simulink model "sim_1_twolink_joint_control_ideal"  (R2021a)
settings: Solver=ode15s  StartTime=0.0  StopTime=15  RelTol=1e-5  EnableMultiTasking=on
values from neighbouring files (symbols this model uses):
  b1 = 0.01    [sim_params.m]    (also in sim_params_force.m)
  b2 = 0.01    [sim_params.m]    (also in sim_params_force.m)
  D = [zeros(n); eye(n)]    [control_comparison_script.m]    (also in gen_twolink_ss.m = reshape([0.0,0.0,0.0,0.0,0.0,0.0,0.0,0.0],[4,2]))
  D_T_Q = D'*Q    [control_comparison_script.m]
  epsilon = 0.1    [control_comparison_script.m]
  g = 9.80665    [sim_params.m]    (also in sim_params_force.m)
  Kd1 = 2.5    [control_comparison_script.m]
  Kd1_grav = 2.5    [control_comparison_script.m]
  Kd1_inv = 12    [control_comparison_script.m]
  Kd1_robust = 7    [control_comparison_script.m]
  Kd2 = 0.5    [control_comparison_script.m]
  Kd2_grav = 0.5    [control_comparison_script.m]
  Kd2_inv = 15    [control_comparison_script.m]
  Kd2_robust = 35    [control_comparison_script.m]
  Klqr = lqr(A,B,Q,R)    [control_comparison_script.m]
  Kp1 = 30    [control_comparison_script.m]
  Kp1_grav = 15    [control_comparison_script.m]
  Kp1_inv = 25    [control_comparison_script.m]
  Kp1_robust = 25    [control_comparison_script.m]
  Kp2 = 7    [control_comparison_script.m]
  Kp2_grav = 3.5    [control_comparison_script.m]
  Kp2_inv = 50    [control_comparison_script.m]
  Kp2_robust = 45    [control_comparison_script.m]
  Kpp = place(A,B,p)    [control_comparison_script.m]
  L1x = 0.3    [sim_params.m]    (also in sim_params_force.m)
  L1y = 0.050    (= 0.05)    [sim_params.m]    (also in sim_params_force.m)
  L1z = 0.05    [sim_params.m]    (also in sim_params_force.m)
  L2x = 0.15    [sim_params.m]    (also in sim_params_force.m = 0.3)
  L2y = 0.05    [sim_params.m]    (also in sim_params_force.m)
  L2z = 0.05    [sim_params.m]    (also in sim_params_force.m)
  m1 = m1*1.25    [control_comparison_script.m]    (also in sim_params.m = 2.775; sim_params_force.m = 2.775)
  m2 = m2*1.25    [control_comparison_script.m]    (also in sim_params.m = 1.3875; sim_params_force.m = 2.775)
  N1 = 100    [control_comparison_script.m]
  N1_grav = 100    [control_comparison_script.m]
  N1_inv = 50    [control_comparison_script.m]
  N1_robust = 50    [control_comparison_script.m]
  N2 = 100    [control_comparison_script.m]
  N2_grav = 100    [control_comparison_script.m]
  N2_inv = 50    [control_comparison_script.m]
  N2_robust = 50    [control_comparison_script.m]
  rho = [1;1]    [control_comparison_script.m]
  theta1_0 = 0    [sim_params.m]    (also in sim_params_force.m = 1.57079632679)
  theta1_dot_0 = 0    [sim_params.m]    (also in sim_params_force.m)
  theta2_0 = 0    [sim_params.m]    (also in sim_params_force.m = -1.57079632679)
  theta2_dot_0 = 0    [sim_params.m]    (also in sim_params_force.m)
  Tsample = 0.001    [sim_params.m]    (also in sim_params_force.m)
undefined symbols (not defined in the file or in its folder): Kd, Ki, Kp, N, sigbuilder_block, X, Y, Z
libraries: pid_lib x12, sm_lib x11, nesl_utility x10, simulink_extras x8, spsFirstOrderFilterLib x4, dspmtrx3 x1
(part 3 of 3)

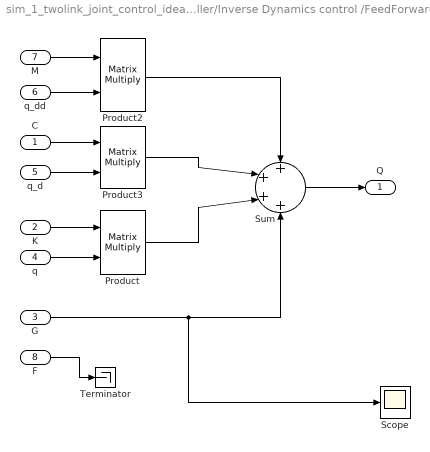
== system sim_1_twolink_joint_control_ideal/Controller/Inverse Dynamics control /FeedForward terms ==
  C : Inport
  K : Inport  Port=2
  G : Inport  Port=3
  q : Inport  Port=4
  q_d : Inport  Port=5
  q_dd : Inport  Port=6
  M : Inport  Port=7
  F : Inport  Port=8
  Product : Product  Multiplication=Matrix(*)
  Product2 : Product  Multiplication=Matrix(*)
  Product3 : Product  Multiplication=Matrix(*)
  Scope : Scope
  Sum : Sum  Inputs=+|+|+|+
  Terminator : Terminator
  Q : Outport
  wires:
  K/1 -> Product/1
  Product/1 -> Sum/3
  Product2/1 -> Sum/1
  Sum/1 -> Q/1
  C/1 -> Product3/1
  Product3/1 -> Sum/2
  M/1 -> Product2/1
  q_dd/1 -> Product2/2
  q/1 -> Product/2
  q_d/1 -> Product3/2
  F/1 -> Terminator/1
  G/1 -> Scope/1, Sum/4

== matlab function sim_1_twolink_joint_control_ideal/Controller/Robust control /Gravity compensation ==
  data: L_1x input; G output; L_2x input; g input; m1 input; m2 input; q1 input; q2 input
function G = G_compensation(L_1x,L_2x,g,m1,m2,q1,q2)
%#codegen

%    This function was generated by the Symbolic Math Toolbox version 8.7.
%    01-Jun-2022 14:38:05

G = [(g.*(L_2x.*m2.*cos(q1+q2)+L_1x.*m1.*cos(q1)+L_1x.*m2.*cos(q1).*2.0))./2.0;
    (L_2x.*g.*m2.*cos(q1+q2))./2.0];

== matlab function sim_1_twolink_joint_control_ideal/Controller/PD-gravity Control /Gravity compensation ==
  data: L_1x input; G output; L_2x input; g input; m1 input; m2 input; q1 input; q2 input
function G = G_compensation(L_1x,L_2x,g,m1,m2,q1,q2)
%#codegen

%    This function was generated by the Symbolic Math Toolbox version 8.7.
%    01-Jun-2022 14:38:05

G = [(g.*(L_2x.*m2.*cos(q1+q2)+L_1x.*m1.*cos(q1)+L_1x.*m2.*cos(q1).*2.0))./2.0;(L_2x.*g.*m2.*cos(q1+q2))./2.0];

== matlab function sim_1_twolink_joint_control_ideal/Controller/Robust control /MATLAB Function ==
  data: z input; w output; epsilon input; rho input
function w = fcn(z, epsilon, rho)
    z_norm = norm(z);
    if z_norm>=epsilon
        w = (rho/z_norm).*z;
    else
        w = (rho/epsilon).*z;
    end

== matlab function sim_1_twolink_joint_control_ideal/Controller/Robust control /simplified_model ==
  data: L_1x input; M_bar output; L_1y input; L_2x input; L_2y input; b1 input; b2 input; m1 input; m2 input; Fv output
function [M_bar,Fv] = simplified_model(L_1x,L_1y,L_2x,L_2y,b1,b2,m1,m2)
%#codegen

%    This function was generated by the Symbolic Math Toolbox version 8.7.
%    17-Jun-2022 16:27:20

M_bar = reshape([(L_1x.^2.*m1)./3.0+L_1x.^2.*m2+(L_1y.^2.*m1)./1.2e+1+(L_2x.^2.*m2)./4.0,0.0,0.0,(m2.*(L_2x.^2.*4.0+L_2y.^2))./1.2e+1],[2,2]);
if nargout > 1
    Fv = reshape([b1,0.0,0.0,b2],[2,2]);
end

== matlab function sim_1_twolink_joint_control_ideal/Controller/Pole Placement+D Control/disturbance_terms ==
  data: L_1x input; d output; L_2x input; g input; m1 input; m2 input; q1 input; q2 input; q1_D input; q2_D input; q1_DD input; q2_DD input
function d = disturbance_terms(L_1x,L_2x,g,m1,m2,q1,q2,q1_D,q2_D,q1_DD,q2_DD)
%#codegen

%    This function was generated by the Symbolic Math Toolbox version 8.7.
%    10-Jun-2022 15:47:18

d = [(g.*(L_2x.*m2.*cos(q1+q2)+L_1x.*m1.*cos(q1)+L_1x.*m2.*cos(q1).*2.0))./2.0+(L_2x.*m2.*q2_DD.*(L_2x+L_1x.*cos(q2).*2.0))./4.0-(L_1x.*L_2x.*m2.*q2_D.^2.*sin(q2))./2.0+L_1x.*L_2x.*m2.*q1_DD.*cos(q2)-L_1x.*L_2x.*m2.*q1_D.*q2_D.*sin(q2);(L_2x.*g.*m2.*cos(q1+q2))./2.0+(L_2x.*m2.*q1_DD.*(L_2x+L_1x.*cos(q2).*2.0))./4.0+(L_1x.*L_2x.*m2.*q1_D.^2.*sin(q2))./2.0];

== matlab function sim_1_twolink_joint_control_ideal/Controller/LQR+D Control/disturbance_terms ==
  data: L_1x input; d output; L_2x input; g input; m1 input; m2 input; q1 input; q2 input; q1_D input; q2_D input; q1_DD input; q2_DD input
function d = disturbance_terms(L_1x,L_2x,g,m1,m2,q1,q2,q1_D,q2_D,q1_DD,q2_DD)
%#codegen

%    This function was generated by the Symbolic Math Toolbox version 8.7.
%    10-Jun-2022 15:47:18

d = [(g.*(L_2x.*m2.*cos(q1+q2)+L_1x.*m1.*cos(q1)+L_1x.*m2.*cos(q1).*2.0))./2.0+(L_2x.*m2.*q2_DD.*(L_2x+L_1x.*cos(q2).*2.0))./4.0-(L_1x.*L_2x.*m2.*q2_D.^2.*sin(q2))./2.0+L_1x.*L_2x.*m2.*q1_DD.*cos(q2)-L_1x.*L_2x.*m2.*q1_D.*q2_D.*sin(q2);(L_2x.*g.*m2.*cos(q1+q2))./2.0+(L_2x.*m2.*q1_DD.*(L_2x+L_1x.*cos(q2).*2.0))./4.0+(L_1x.*L_2x.*m2.*q1_D.^2.*sin(q2))./2.0];

== matlab function sim_1_twolink_joint_control_ideal/Robot/SIMULINK_MODEL/MCKGQ ==
  data: L_1x input; M output; L_1y input; L_2x input; L_2y input; b1 input; b2 input; g input; m1 input; m2 input; q1 input; q2 input; q1_D input; q2_D input; tau1 input; tau2 input; C output; K output; G output; Q output
function [M,C,K,G,Q] = MCKGQ(L_1x,L_1y,L_2x,L_2y,b1,b2,g,m1,m2,q1,q2,q1_D,q2_D,tau1,tau2)
%#codegen

%    This function was generated by the Symbolic Math Toolbox version 8.7.
%    30-May-2022 13:59:37

M = reshape([(L_1x.^2.*m1)./3.0+L_1x.^2.*m2+(L_1y.^2.*m1)./1.2e+1+(L_2x.^2.*m2)./4.0+L_1x.*L_2x.*m2.*cos(q2),(L_2x.*m2.*(L_2x+L_1x.*cos(q2).*2.0))./4.0,(L_2x.*m2.*(L_2x+L_1x.*cos(q2).*2.0))./4.0,(m2.*(L_2x.^2.*4.0+L_2y.^2))./1.2e+1],[2,2]);
if nargout > 1
    C = reshape([-L_1x.*L_2x.*m2.*q2_D.*sin(q2),(L_1x.*L_2x.*m2.*q1_D.*sin(q2))./2.0,L_1x.*L_2x.*m2.*q2_D.*sin(q2).*(-1.0./2.0),0.0],[2,2]);
end
if nargout > 2
    K = reshape([0.0,0.0,0.0,0.0],[2,2]);
end
if nargout > 3
    G = [(g.*(L_2x.*m2.*cos(q1+q2)+L_1x.*m1.*cos(q1)+L_1x.*m2.*cos(q1).*2.0))./2.0;(L_2x.*g.*m2.*cos(q1+q2))./2.0];
end
if nargout > 4
    Q = [tau1-b1.*q1_D;tau2-b2.*q2_D];
end

== matlab function sim_1_twolink_joint_control_ideal/Robot/SIMULINK_MODEL/MATLAB Function1 ==
  data: M input; the_cond output
function the_cond = COND(M)
%#codegen

the_cond = cond(M);

end

== matlab function sim_1_twolink_joint_control_ideal/Controller/PD-feedforward-gravity Control/Gravity compensation ==
  data: L_1x input; G output; L_2x input; g input; m1 input; m2 input; q1 input; q2 input
function G = G_compensation(L_1x,L_2x,g,m1,m2,q1,q2)
%#codegen

%    This function was generated by the Symbolic Math Toolbox version 8.7.
%    01-Jun-2022 14:38:05

G = [(g.*(L_2x.*m2.*cos(q1+q2)+L_1x.*m1.*cos(q1)+L_1x.*m2.*cos(q1).*2.0))./2.0;(L_2x.*g.*m2.*cos(q1+q2))./2.0];

== matlab function sim_1_twolink_joint_control_ideal/Controller/Inverse Dynamics control /MCKGQ ==
  data: L_1x input; M output; L_1y input; L_2x input; L_2y input; b1 input; b2 input; g input; m1 input; m2 input; q1 input; q2 input; q1_D input; q2_D input; tau1 input; tau2 input; C output; K output; G output; Q output
function [M,C,K,G,Q] = MCKGQ(L_1x,L_1y,L_2x,L_2y,b1,b2,g,m1,m2,q1,q2,q1_D,q2_D,tau1,tau2)
%#codegen

%    This function was generated by the Symbolic Math Toolbox version 8.7.
%    30-May-2022 13:59:37

M = reshape([(L_1x.^2.*m1)./3.0+L_1x.^2.*m2+(L_1y.^2.*m1)./1.2e+1+(L_2x.^2.*m2)./4.0+L_1x.*L_2x.*m2.*cos(q2),(L_2x.*m2.*(L_2x+L_1x.*cos(q2).*2.0))./4.0,(L_2x.*m2.*(L_2x+L_1x.*cos(q2).*2.0))./4.0,(m2.*(L_2x.^2.*4.0+L_2y.^2))./1.2e+1],[2,2]);
if nargout > 1
    C = reshape([-L_1x.*L_2x.*m2.*q2_D.*sin(q2),(L_1x.*L_2x.*m2.*q1_D.*sin(q2))./2.0,L_1x.*L_2x.*m2.*q2_D.*sin(q2).*(-1.0./2.0),0.0],[2,2]);
end
if nargout > 2
    K = reshape([0.0,0.0,0.0,0.0],[2,2]);
end
if nargout > 3
    G = [(g.*(L_2x.*m2.*cos(q1+q2)+L_1x.*m1.*cos(q1)+L_1x.*m2.*cos(q1).*2.0))./2.0;(L_2x.*g.*m2.*cos(q1+q2))./2.0];
end
if nargout > 4
    Q = [tau1-b1.*q1_D;tau2-b2.*q2_D];
end
